simulink model "Task_8_Linear_Rhose"  (R2018a)
settings: Solver=VariableStepAuto  StartTime=0.0  StopTime=10.0  MaxStep=0.001  RelTol=1e-3
libraries: simulink x2
settings Model: Creator=HP  LastModifiedBy=HP

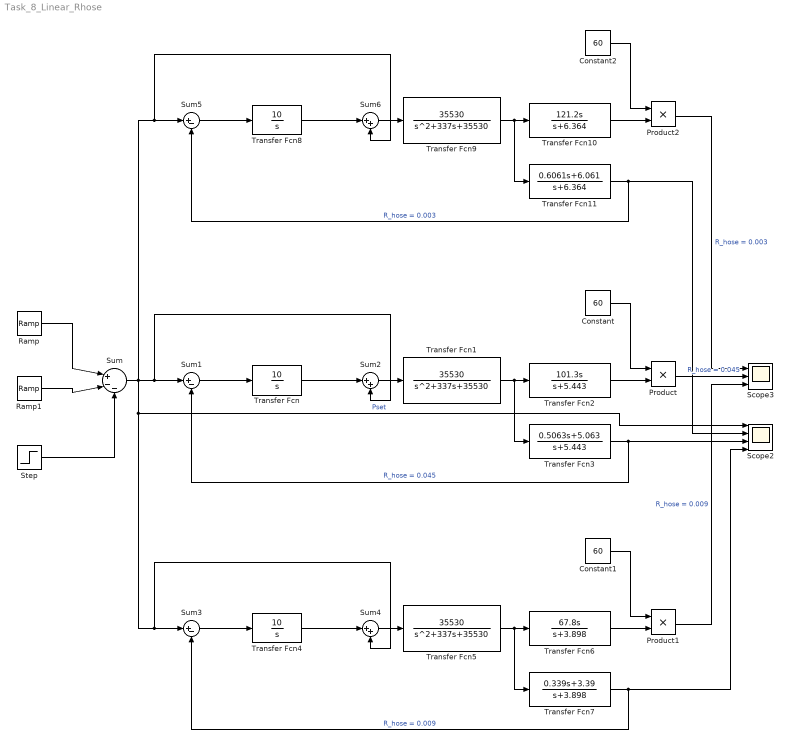
== system Task_8_Linear_Rhose ==
  Constant : Constant  Value=60
  Constant1 : Constant  Value=60
  Constant2 : Constant  Value=60
  Product : Product
  Product1 : Product
  Product2 : Product
  Ramp : simulink/Sources/Ramp  slope=64.9351  start=1  InitialOutput=0
  Ramp1 : simulink/Sources/Ramp  slope=64.9531  start=1.231  InitialOutput=0
  Scope2 : Scope  NumInputPorts=4
  Scope3 : Scope  NumInputPorts=3
  Step : Step  Time=5  After=15  SampleTime=0
  Sum : Sum  Inputs=|+--
  Sum1 : Sum  Inputs=|+-
  Sum2 : Sum  Inputs=|++
  Sum3 : Sum  Inputs=|+-
  Sum4 : Sum  Inputs=|++
  Sum5 : Sum  Inputs=|+-
  Sum6 : Sum  Inputs=|++
  Transfer Fcn : TransferFcn  Numerator=[10]  Denominator=[1 0]
  Transfer Fcn1 : TransferFcn  Numerator=[35530]  Denominator=[1 337 35530]
  Transfer Fcn10 : TransferFcn  Numerator=[121.2 0]  Denominator=[1 6.364]
  Transfer Fcn11 : TransferFcn  Numerator=[0.6061 6.061]  Denominator=[1 6.364]
  Transfer Fcn2 : TransferFcn  Numerator=[101.3 0]  Denominator=[1 5.443]
  Transfer Fcn3 : TransferFcn  Numerator=[0.5063 5.063]  Denominator=[1 5.443]
  Transfer Fcn4 : TransferFcn  Numerator=[10]  Denominator=[1 0]
  Transfer Fcn5 : TransferFcn  Numerator=[35530]  Denominator=[1 337 35530]
  Transfer Fcn6 : TransferFcn  Numerator=[67.8 0]  Denominator=[1 3.898]
  Transfer Fcn7 : TransferFcn  Numerator=[0.339 3.39]  Denominator=[1 3.898]
  Transfer Fcn8 : TransferFcn  Numerator=[10]  Denominator=[1 0]
  Transfer Fcn9 : TransferFcn  Numerator=[35530]  Denominator=[1 337 35530]
  wires:
  Transfer Fcn4/1 -> Sum4/1
  Step/1 -> Sum/3
  Transfer Fcn8/1 -> Sum6/1
  Product/1 -> Scope3/2  "R_hose = 0.045"
  Transfer Fcn1/1 -> Transfer Fcn3/1, Transfer Fcn2/1
  Product2/1 -> Scope3/1  "R_hose = 0.003"
  Transfer Fcn10/1 -> Product2/2
  Constant1/1 -> Product1/1
  Transfer Fcn3/1 -> Scope2/3, Sum1/2  "R_hose = 0.045"
  Transfer Fcn2/1 -> Product/2
  Sum3/1 -> Transfer Fcn4/1
  Sum2/1 -> Transfer Fcn1/1
  Transfer Fcn6/1 -> Product1/2
  Transfer Fcn7/1 -> Scope2/4, Sum3/2  "R_hose = 0.009"
  Sum4/1 -> Transfer Fcn5/1
  Transfer Fcn9/1 -> Transfer Fcn11/1, Transfer Fcn10/1
  Ramp/1 -> Sum/1
  Transfer Fcn/1 -> Sum2/1
  Transfer Fcn5/1 -> Transfer Fcn7/1, Transfer Fcn6/1
  Sum6/1 -> Transfer Fcn9/1
  Sum5/1 -> Transfer Fcn8/1
  Product1/1 -> Scope3/3  "R_hose = 0.009"
  Sum1/1 -> Transfer Fcn/1
  Ramp1/1 -> Sum/2
  Transfer Fcn11/1 -> Scope2/2, Sum5/2  "R_hose = 0.003"
  Constant2/1 -> Product2/1
  Constant/1 -> Product/1
  Sum/1 -> Scope2/1, Sum4/2, Sum3/1, Sum6/2, Sum5/1, Sum2/2, Sum1/1  "Pset"
